simulink model "controllo_test"  (R2020a)
settings: Solver=VariableStepAuto  StartTime=0.0  StopTime=100  RelTol=1e-3
values from neighbouring files (symbols this model uses):
  a = 0.35    [data.m]    (also in geodetic2nedS.m = 6378137)
  a1 = rho * D^4 * alpha1    (= 0.000388302366464)    [data.m]
  a2 = -rho * D^3 * alpha2 * (1 - omega)    (= 0.0037030698432)    [data.m]
  AHRS_bias = [0 0 0]    [data.m]
  AHRS_sample_time = 1/50    (= 0.02)    [data.m]
  AHRS_var = ([1 1 2] * pi/180).^2    [data.m]
  alpha1 = 0.0113    [data.m]
  alpha2 = -0.0091    [data.m]
  c = son2(1)    [Sonar_id.m]    (also in data.m = 0.19)
  current = [seaCurrent; 0; 0; 0]    [data.m]
  D = 0.076    [data.m]
  dead_zone_limit = 31.5    [data.m]
  DVL_sample_t = 1/12    (= 0.0833333333333)    [data.m]
  DVL_var1 = 0.005^2    (= 2.5e-05)    [data.m]
  DVL_var2 = 0.015^2    (= 0.000225)    [data.m]
  DVL_var3 = 0.023^2    (= 0.000529)    [data.m]
  gps_sample_t = 1    [data.m]
  H = eye(3)    [data.m]    (also in navigation_data.m)
  IMU_sample_time = 1/100    (= 0.01)    [data.m]
  initial = []    [data.m]
  INSP = unicode2native(inspectionDirection)    [data.m]
  Ki_bodypos1 = 0    [parametri_PID.m]
  Ki_bodypos2 = 0    [parametri_PID.m]
  Ki_bodypos3 = 0    [parametri_PID.m]
  Ki_bodypos4 = 0    [parametri_PID.m]
  Ki_bodypos5 = 0    [parametri_PID.m]
  Ki_depth1 = 0    [parametri_PID.m]
  Ki_depth2 = 0    [parametri_PID.m]
  Ki_depth3 = 0    [parametri_PID.m]
  Ki_depth4 = 0    [parametri_PID.m]
  Ki_depth5 = 0    [parametri_PID.m]
  Ki_latvel1 = 0    [parametri_PID.m]
  Ki_latvel2 = 0    [parametri_PID.m]
  Ki_latvel3 = 0    [parametri_PID.m]
  Ki_latvel4 = 0    [parametri_PID.m]
  Ki_latvel5 = 0    [parametri_PID.m]
  Ki_P1 = 0    [parametri_PID.m]
  Ki_P2 = 0    [parametri_PID.m]
  Ki_P3 = 0    [parametri_PID.m]
  Ki_P4 = 0    [parametri_PID.m]
  Ki_P5 = 0    [parametri_PID.m]
  Ki_R1 = 0    [parametri_PID.m]
  Ki_R2 = 0    [parametri_PID.m]
  Ki_R3 = 0    [parametri_PID.m]
  Ki_R4 = 0    [parametri_PID.m]
  Ki_R5 = 0    [parametri_PID.m]
  Ki_rel_or1 = 0    [parametri_PID.m]
  Ki_rel_or2 = 0    [parametri_PID.m]
  Ki_rel_or3 = 0    [parametri_PID.m]
  Ki_rel_or4 = 0    [parametri_PID.m]
  Ki_rel_or5 = 0    [parametri_PID.m]
  Ki_reldist1 = 0    [parametri_PID.m]
  Ki_reldist2 = 0    [parametri_PID.m]
  Ki_reldist3 = 0    [parametri_PID.m]
  Ki_reldist4 = 0    [parametri_PID.m]
  Ki_reldist5 = 0    [parametri_PID.m]
  Ki_surge1 = 0    [parametri_PID.m]
  Ki_surge2 = 0    [parametri_PID.m]
  Ki_surge3 = 0    [parametri_PID.m]
  Ki_surge4 = 0    [parametri_PID.m]
  Ki_surge5 = 0    [parametri_PID.m]
  Ki_yaw1 = 0    [parametri_PID.m]
  Ki_yaw2 = 0    [parametri_PID.m]
  Ki_yaw3 = 0    [parametri_PID.m]
  Ki_yaw4 = 0    [parametri_PID.m]
  Ki_yaw5 = 0    [parametri_PID.m]
  Kp_bodypos1 = 0    [parametri_PID.m]
  Kp_bodypos2 = 2    [parametri_PID.m]
  Kp_bodypos3 = 2    [parametri_PID.m]
  Kp_bodypos4 = 2    [parametri_PID.m]
  Kp_bodypos5 = 2    [parametri_PID.m]
  Kp_depth1 = 0    [parametri_PID.m]
  Kp_depth2 = 2    [parametri_PID.m]
  Kp_depth3 = 2    [parametri_PID.m]
  Kp_depth4 = 2    [parametri_PID.m]
  Kp_depth5 = 2    [parametri_PID.m]
  Kp_latvel1 = 0    [parametri_PID.m]
  Kp_latvel2 = 2    [parametri_PID.m]
  Kp_latvel3 = 2    [parametri_PID.m]
  Kp_latvel4 = 2    [parametri_PID.m]
  Kp_latvel5 = 2    [parametri_PID.m]
  Kp_P1 = 0    [parametri_PID.m]
  Kp_P2 = 2    [parametri_PID.m]
  Kp_P3 = 2    [parametri_PID.m]
  Kp_P4 = 2    [parametri_PID.m]
  Kp_P5 = 2    [parametri_PID.m]
  Kp_R1 = 0    [parametri_PID.m]
  Kp_R2 = 2    [parametri_PID.m]
  Kp_R3 = 2    [parametri_PID.m]
  Kp_R4 = 2    [parametri_PID.m]
  Kp_R5 = 2    [parametri_PID.m]
  Kp_rel_or1 = 0    [parametri_PID.m]
  Kp_rel_or2 = 2    [parametri_PID.m]
  Kp_rel_or3 = 2    [parametri_PID.m]
  Kp_rel_or4 = 2    [parametri_PID.m]
  Kp_rel_or5 = 2    [parametri_PID.m]
  Kp_reldist1 = 0    [parametri_PID.m]
  Kp_reldist2 = 2    [parametri_PID.m]
  Kp_reldist3 = 2    [parametri_PID.m]
  Kp_reldist4 = 2    [parametri_PID.m]
  Kp_reldist5 = 2    [parametri_PID.m]
  Kp_surge1 = 0    [parametri_PID.m]
  Kp_surge2 = 2    [parametri_PID.m]
  Kp_surge3 = 2    [parametri_PID.m]
  Kp_surge4 = 2    [parametri_PID.m]
  Kp_surge5 = 2    [parametri_PID.m]
  Kp_yaw1 = 0.6*6    (= 3.6)    [parametri_PID.m]
  Kp_yaw2 = 2    [parametri_PID.m]
  Kp_yaw3 = 2    [parametri_PID.m]
  Kp_yaw4 = 2    [parametri_PID.m]
  Kp_yaw5 = 2    [parametri_PID.m]
  M = M_rb + M_a    [Masse.m]
  M_inv = inv(M)    [Masse.m]
  n_max = 340    [data.m]
  num_cycle = 5    [data.m]    (also in navigation_data.m)
  omega = 0.1    [data.m]
  ps_sample_t = 0.02    [data.m]
  ps_var = (5000/3)^2    (= 2777777.77778)    [data.m]
  pylonCenter = [ 43.723046 ... (first row only)    [missionB.m]
  pylonRadius = 10    [missionB.m]
  ... (+3 more)
undefined symbols (not defined in the file or in its folder): arrival_point, DiscIntNeverNeededParam, Kd_bodypos2, Kd_bodyposy2, Kd_dist_mis2, Kd_surge2, Kd_yaw1, Ki_bodyposy2, Ki_dist_mis2, Kp_dist_mis2, s_data
libraries: simulink x8
(part 4 of 4)

== matlab function controllo_test/Env. & Sensor Model/DVL SENSOR/MATLAB Function ==
  data: ni input; niDVL output; c parameter
function niDVL = traslation(ni, c)
%Calcola la velocità in terna DVL

S = [0,-ni(6),ni(5); 
    ni(6),0,-ni(4); 
    -ni(5),ni(4),0];
p = [0;0;c];
niDVL = ni(1:3,1)+S*p;        %Formula fondamentale della cinematica

== matlab function controllo_test/Vehicle Model/Model Vehicle/D ==
  data: ni_r input; F_d output; rho input
function F_d = D_forces(ni_r, rho)
    ni_lin = ni_r(1:3);
    ni_ang = ni_r(4:6);
    a = 0.35;
    b = a;
    c = 0.19;
    A_ab = pi*a*b;      % moto lin lungo z; rotatorio intorno a x e y
    A_bc = pi*b*c;      % moto lin lungo x; rotatorio intorno a z
    A_ac = pi*a*c;      % moto lin lungo y
%     C_d  =  0.0489;
%     D_coeff = -1/2*rho*C_d*diag([A_bc, A_ac, A_ab, A_bc, A_ac, A_ab]);
%     F_d = D_coeff*(abs(ni_r).*ni_r);
    visc = 0.001;       % Pa*s (per una temperatura di 20° e rho = 1030)
    vmax = 0.3;
    Di = 0.7;
    Re = Di/(visc/rho)*vmax; % Re = 2*1e5
    Cd = 0.49;
    rm_z = 4*c/(3*pi);
    rm_xy = 4*a/(3*pi);
    D_lin = -1/2*rho*Cd*diag([A_bc, A_ac, A_ab])*(abs(ni_lin).*ni_lin);
    D_ang = -1/2*rho*Cd*diag([rm_xy^3*A_ab, rm_xy^3*A_ab, rm_z^3*A_bc])*(abs(ni_ang).*ni_ang);
    F_d = [D_lin; D_ang];
end

== matlab function controllo_test/Env. & Sensor Model/DVL SENSOR/MATLAB Function2 ==
  data: v input; flag output
function flag  = vel_module(v)
%Calcola il modulo della velocità per controllare le condizioni di
%funzionamento del DVL

mod = sqrt((v(1))^2+(v(2))^2+(v(3))^2);

%Da datasheet, se la velocità è superiore ai 9 m/s il sensore non funziona bene
if mod > 9
    flag = 0;
else
    flag = 1;
end
end

== matlab function controllo_test/Controller/AVVICINAMENTO/J2_inv ==
  data: tau_roll input; tau_or_body output; tau_pitch input; tau_yaw input; est_state input
function tau_or_body = fcn(tau_roll,tau_pitch,tau_yaw,est_state)
theta=est_state(1);
phi=est_state(2);
tau_or=[tau_roll;tau_pitch;tau_yaw];
J2_inv = [1       0          -sin(theta); 
         0   cos(phi)  cos(theta)*sin(phi);
         0  -sin(phi)  cos(theta)*cos(phi)];
tau_or_body=J2_inv*tau_or;
end

== matlab function controllo_test/Controller/GEODETIC2NED2/GEODETIC2NED1/MATLAB Function ==
  data: lat input; pos_s_Ned output; lon input
function pos_s_Ned = fcn(lat,lon)
coder.extrinsic('wgs84Ellipsoid','geodetic2ned');
pylonCenter = [43.723046;10.396635];
initPoint = [ 43.722984;10.396204;0];
hOrigin=0;
pos_s_Ned=zeros(3,1);
wgs84=wgs84Ellipsoid('meter');
lat0=pylonCenter(1);
lon0=pylonCenter(2);
h=initPoint(3);
h0=hOrigin;
[xs_N,ys_E,zs_D]=geodetic2ned(lat,lon,h,lat0,lon0,h0,wgs84);
pos_s_Ned=[xs_N,ys_E,zs_D]';
end

== matlab function controllo_test/Env. & Sensor Model/Pressure sensor/MATLAB Function2 ==
  data: h input; p output; rho parameter
function p = pressure(h, rho)
%Calcola la pressione a partire dalla profondità

g = 9.81;                        %accelerazione gravitazionale
p = rho*g*h;
end

== matlab function controllo_test/Env. & Sensor Model/Pressure sensor/MATLAB Function3 ==
  data: orient input; p input; h output; rho parameter; c parameter
function h = depth( orient,  p, rho, c)
%Calcola la profondità misurata dal sensore

phi = orient(1);
theta = orient(2);
psi = orient(3);
Rx_phi = [1 0 0; 0 cos(phi) -sin(phi); 0 sin(phi) cos(phi)];
Ry_theta = [cos(theta) 0 sin(theta); 0 1 0; -sin(theta) 0 cos(theta)];
Rz_psi = [cos(psi) -sin(psi) 0; sin(psi) cos(psi) 0; 0 0 1];

R = Rz_psi*Ry_theta*Rx_phi;
g = 9.81;
cNED = R*[0;0;c];                            %Vettore posizione dell'AUV in terna body riportato in terna NED
h = p/(rho*g)+cNED(3);                       %Il profondimetro è installato sulla pancia dell'AUV, lungo l'asse z
end

== matlab function controllo_test/Controller/GEODETIC2NED3/GEODETIC2NED/MATLAB Function ==
  data: lat input; lon input; pos_Ned output
function pos_Ned = fcn (lat,lon)
coder.extrinsic('wgs84Ellipsoid','geodetic2ned');
pylonCenter = [43.723046;10.396635];
initPoint = [ 43.722984;10.396204;0];
hOrigin=0;
pos_Ned=zeros(3,1)
wgs84=wgs84Ellipsoid('meter')
h=initPoint(3)
lat0=pylonCenter(1)
lon0=pylonCenter(2)
h0=hOrigin
[x_N,y_E,z_D]=geodetic2ned(lat,lon,h,lat,lon,h,wgs84); %TOFIX
pos_Ned=[x_N,y_E,z_D]'
end

== matlab function controllo_test/Controller/IMMERSIONE//RISALITA/J2_inv ==
  data: tau_roll input; tau_or_body output; tau_pitch input; tau_yaw input; est_state input
function tau_or_body = fcn(tau_roll,tau_pitch,tau_yaw,est_state)
theta=est_state(1);
phi=est_state(2);
tau_or=[tau_roll;tau_pitch;tau_yaw];
J2_inv = [1       0          -sin(theta); 
         0   cos(phi)  cos(theta)*sin(phi);
         0  -sin(phi)  cos(theta)*cos(phi)];
tau_or_body=J2_inv*tau_or;
end

== matlab function controllo_test/Env. & Sensor Model/Sonar sensor/MATLAB Function ==
  data: xNorth input; s output; yEast input; zDown input; roll input; pitch input; yaw input; pylonRadius parameter; s_data parameter
function s = Sonar_ideal(xNorth,yEast,zDown,roll,pitch,yaw,pylonRadius, s_data)

coder.extrinsic('Sonar_id');

s_data.num = 5;
s = zeros(s_data.num,1);

s = Sonar_id(xNorth,yEast,zDown,roll,pitch,yaw,pylonRadius,s_data);

== matlab function controllo_test/Vehicle Model/Model Vehicle/C ==
  data: ni_r input; F_c output; M input
function F_c = C(ni_r, M)
    ni = ni_r;
    M11 = M(1:3,1:3);
    M22 = M(4:6,4:6);
    ni1 = ni(1:3);
    ni2 = ni(4:6);
    C11 = zeros(3,3);
    s1 = M11*ni1;
    C12 = - [0 -s1(3) s1(2); s1(3) 0 -s1(1); -s1(2) s1(1) 0];
    C21 = C12;
    s2 = M22*ni2;
    C22 = - [0 -s2(3) s2(2); s2(3) 0 -s2(1); -s2(2) s2(1) 0];
    F_c = [C11 C12; C21 C22]*ni_r;
end

== matlab function controllo_test/Env. & Sensor Model/Sonar sensor/MATLAB Function1 ==
  data: s_in input; s_out output; depth input; error input; flag output; s_data parameter
function [s_out,flag] = Sonar_lim(s_in,depth,error,s_data)
%SONAR_lim
%     [s_out,flag] = Sonar_id[s,error]
%
% Returns the sonar output considering the sensors limitations, but not
% taking into account the bias and error.
%
% flag signals that the corresponding sensor output is affected by
% problems:
% flag += 0     ==>     No errors
% flag += 1     ==>     Under minimum detectable range
% flag += 2     ==>     Over maximum detectable range
% flag += 4     ==>     Over maximum depth
% flag += 8     ==>     Other errors
%
% error is a boolean variable which, when true, sets the flag to += 8

s_data.num = 5;

flag = zeros(s_data.num,1);

s_out = s_in;

for i=1:s_data.num
    if s_in(i) < s_data.minrng
    % Too close
        flag(i) = flag(i)+1;
        s_out(i) = s_data.minrng;
    end
    
    if ( s_in(i) > s_data.maxrng || isnan(s_in(i)) )
    % Too far
        flag(i) = flag(i)+2;
        s_out(i) = NaN;
    end
    
    if depth > s_data.maxdpt
    % Over max depth
        flag(i) = flag(i)+4;
        s_out(i) = NaN;
    end
    
    if error(i) > 0
    % General error flag
        flag(i) = flag(i) + error(i);
        s_out(i) = NaN;
    end
end

end

== matlab function controllo_test/Controller/MATLAB Function1 ==
  data: STATE input; EN output; dist_mis input; yaw_err input; depth_err input; INSP input string
function EN = fcn(STATE,dist_mis,yaw_err,depth_err, INSP)

%EN(1)= bodypos_err
%EN(2)= rel_dist_err
%EN(3)=surge_err
%EN(4)= latvel_err
%EN(5)=depth_err
%EN(6)= RP_err
%EN(7)= rel_or_err
%EN(8)= yaw_err

EN=zeros(1,8)';

if (STATE == 101)
    EN(8)=1;
end
%avvicinamento pilone
if (STATE== 102)
    EN(8)=1;
    EN(3)=1;
    if (STATE==102) && dist_mis<=3.63
        EN(8)=1;
        EN(1)=1;
        EN(3)=0;
    end
end
%rotazione attorno al pilone in superficie
if (STATE == 103)
    EN(2)=1;
    EN(7)=1;
    EN(4)=1;    
    if (yaw_err<=10)
        EN(4)=0;
        EN(8)=1;
        EN(2)=1;
        EN(7)=0;
    end
end
%unicodestr = native2unicode(INSP);
s1=INSP;
s2='vertical';
CMP=strcmp(s1,s2);
if (CMP == 1) %inizio ispezione verticale
    if (STATE==201) 
        EN(2)=1;
        EN(5)=1;
        EN(7)=1;
        EN(6)=1;
        if(depth_err<=3) %stacco i thrusters che controllano la depth
            EN(2)=1;
            EN(7)=1;
            EN(5)=0;
            EN(6)=1;   
        end
    end
    if(STATE==202) && (depth_err<0.2) %controllo di velocità laterale
        EN(2)=1;
        EN(4)=1;
        EN(5)=1;
        EN(6)=1;
        EN(7)=1;
        if(yaw_err<=10) %switch su controllo di posizione
            EN(8)=1;
            EN(2)=1;
            EN(7)=0;
            EN(4)=0; 
            EN(5)=1;
            EN(6)=1;
        end
    end  %fine ispezione verticale
else
    if (STATE==202) && (depth_err<0.2) % inizio ispezione orizzontale
        EN(2)=1;
        EN(5)=1;
        EN(4)=1;  
        EN(7)=1;  
        EN(6)=1;
        if(yaw_err<=10) %switch su controllo di yaw
            EN(8)=1;
            EN(2)=1;
            EN(7)=0; 
            EN(4)=0;
            EN(5)=1;
            EN(6)=1;
        end
    end
    if (STATE==201) %transetto verticale in isp. orizzontale
        EN(2)=1;
        EN(7)=1;
        EN(5)=1;
        EN(6)=1;   
    end 
end     %fine ispezione orizzontale
%fase di immersione   
if(STATE==104)
   EN(2)=1;
   EN(7)=1;
   EN(5)=1;
   EN(6)=1;
   if(depth_err<=3) %stacco i thrusters che controllano la depth
        EN(2)=1;
        EN(7)=1;
        EN(5)=0;
        EN(6)=1;   
   end
end
%fase di risalita
if(STATE==401)
   EN(2)=1;
   EN(7)=1;
   EN(5)=1;
   EN(6)=1;
end   
   
%fase di errore e fine missione
if(STATE == 500) || (STATE == 999)% lascio così poichè in caso di errore
   EN=zeros(1,8)';               % comunque spegnamo tutti i segnali e
                                % lo facciamo risalire attraverso i 4N
end
end

== matlab function controllo_test/Env. & Sensor Model/geodetic2NED1 ==
  data: x output; u input; y output; z output; pylonCenter parameter
function [x, y, z] = fcn(u, pylonCenter)


lat_origin = pylonCenter(1);
lon_origin= pylonCenter(2);
h_origin = pylonCenter(3);

lat=u(1);
lon=u(2);
h=u(3);


[xNorth, yEast, zDown] = geodetic2nedS(lat, lon, h, lat_origin, lon_origin, h_origin);

x = xNorth;
y = yEast;
z = h;

== matlab function controllo_test/Controller/NED2BODY ==
  data: eta1_dot input; mi1 output; phi input; theta input; psi input
function mi1 = fcn(eta1_dot,phi,theta,psi)
Rx_phi=[1 0 0;0 cos(phi) -sin(phi);0 sin(phi) cos(phi)];
Ry_theta=[cos(theta) 0 sin(theta);0 1 0;-sin(theta) 0 cos(theta)];
Rz_psi=[cos(psi) -sin(psi) 0;sin(psi) cos(psi) 0;0 0 1];
J1=Rx_phi*Ry_theta*Rz_psi;
mi1 =J1^-1*eta1_dot;

== matlab function controllo_test/Controller/NED2BODY1 ==
  data: abspos_err input; bodypos_err output; phi input; theta input; psi input
function bodypos_err = fcn(abspos_err,phi,theta,psi)
Rx_phi=   [1      0        0;
           0   cos(phi) -sin(phi);
           0   sin(phi) cos(phi)];
    
Ry_theta=[cos(theta) 0  sin(theta);
              0      1      0;
         -sin(theta) 0  cos(theta)];
     
Rz_psi=  [cos(psi) -sin(psi)  0;
          sin(psi)  cos(psi)  0;
           0           0      1];
       
J1=Rx_phi*Ry_theta*Rz_psi;
bodypos_err=J1^-1*abspos_err

== matlab function controllo_test/Controller/POSIZIONAMENTO/J2_inv ==
  data: tau_roll input; tau_or_body output; tau_pitch input; tau_yaw input; est_state input
function tau_or_body = fcn(tau_roll,tau_pitch,tau_yaw,est_state)
theta=est_state(1);
phi=est_state(2);
tau_or=[tau_roll;tau_pitch;tau_yaw];
J2_inv = [1       0          -sin(theta); 
         0   cos(phi)  cos(theta)*sin(phi);
         0  -sin(phi)  cos(theta)*cos(phi)];
tau_or_body=J2_inv*tau_or;
end

== matlab function controllo_test/Controller/ROTAZIONE IN PROFONDITA'/J2_inv ==
  data: tau_roll input; tau_or_body output; tau_pitch input; tau_yaw input; est_state input
function tau_or_body = fcn(tau_roll,tau_pitch,tau_yaw,est_state)
theta=est_state(1);
phi=est_state(2);
tau_or=[tau_roll;tau_pitch;tau_yaw];
J2_inv = [1       0          -sin(theta); 
         0   cos(phi)  cos(theta)*sin(phi);
         0  -sin(phi)  cos(theta)*cos(phi)];
tau_or_body=J2_inv*tau_or;
end

== matlab function controllo_test/Controller/ROTAZIONE IN SUPERFICIE/J2_inv ==
  data: tau_roll input; tau_or_body output; tau_pitch input; tau_yaw input; est_state input
function tau_or_body = fcn(tau_roll,tau_pitch,tau_yaw,est_state)
theta=est_state(1);
phi=est_state(2);
tau_or=[tau_roll;tau_pitch;tau_yaw];
J2_inv = [1       0          -sin(theta); 
         0   cos(phi)  cos(theta)*sin(phi);
         0  -sin(phi)  cos(theta)*cos(phi)];
tau_or_body=J2_inv*tau_or;
end

== matlab function controllo_test/Vehicle Model/Model Vehicle/grav ==
  data: rho input; eta input; F_g output
function F_g = grav(rho, eta)
    eta2 = eta(4:6);
    g = 9.81;   
    a = 0.35;
    b = a;
    c = 0.19;
    massa = 100;
    if eta(3) >= c
       V = 4/3*pi*a*b*c;
    else
       V = 4/3*pi*a*b*c - (pi*a*b/(3*c^2))*((eta(3)-c)^2)*(3*c - abs(eta(3) - c)); 
    end
    W = massa*g;
    B = rho*V*g;
    J = Jac(eta2);
    J1 = J(1:3,1:3);
    J2 = J(4:6,4:6);
    f_g = inv(J1)*[0; 0; W];
    f_b = inv(J1)*[0; 0; -B];
    r_g = [0; 0; 0];
    r_b = [0; 0; -c/2];
    %TODO: inserire un contributo nullo di forza quando siamo a galla (?)
%     if eta(3) < 0
%        F_g = [0; 0; 0; 0; 0; 0];
%     else
    F_g = -[f_g + f_b; cross(r_g,f_g) + cross(r_b,f_b)];
%     end
end

== matlab function controllo_test/Controller/T2n/MATLAB Function ==
  data: Tdes input; n output
function n  = fcn(Tdes)
n=zeros(1,7)';
a1=0.000388302366464000;
%assunzione modello a bassa velocità
for i=1:1:7
       n(i)=sign(Tdes(i))*sqrt((abs(Tdes(i))/a1));  
end
end

== matlab function controllo_test/Controller/Tau2T/Tau2T ==
  data: tau_des input; T output
function T= fcn(tau_des)
p1 = [0 -0.25 0]';
p2 = [0 0.25 0]';
p3 = [-0.25 0 0]';
p4 = [0.25 0 0]';
p5 = [-0.15 -0.15 0]';
p6 = [-0.15 0.15 0]';
p7 = [0.15 0 0]';

t1 = [1 0 0]';
t2 = t1;
t3 = [0 1 0]';
t4 = -t3;
t5 = [0 0 1]';
t6 = t5;
t7 = t5;

B1 = [t1; cross(p1,t1)];
B2 = [t2; cross(p2,t2)];
B3 = [t3; cross(p3,t3)];
B4 = [t4; cross(p4,t4)];
B5 = [t5; cross(p5,t5)];
B6 = [t6; cross(p6,t6)];
B7 = [t7; cross(p7,t7)];
B = [B1 B2 B3 B4 B5 B6 B7];

Bpinv=pinv(B);
T = Bpinv*tau_des;

end

== matlab function controllo_test/Controller/Tau2T/Tau_des ENABLE ==
  data: STATE input; tau_des output; tau1 input; tau2 input; tau3 input; tau4 input; tau5 input
function tau_des= fcn(STATE,tau1,tau2,tau3,tau4,tau5)
tau_des= zeros(1,6)';
if (STATE==101)
    tau_des=tau1;
end
if (STATE==102)
    tau_des=tau2;
end
if (STATE==103)
    tau_des= tau3;
end
if (STATE== 201|| STATE==104||STATE==401)
    tau_des=tau4;
end
if (STATE== 202)
    tau_des=tau5;
end
if (STATE==500 || STATE== 999)
    tau_des=zeros(1,6)';
end
end

== matlab function controllo_test/Controller/wrapTopi ==
  data: u input; y output
function y = fcn(u)
coder.extrinsic('wrapToPi');
y=0;
y = wrapToPi(u);
end

== matlab function controllo_test/Controller/wrapTopi1 ==
  data: u input; y output
function y = fcn(u)
coder.extrinsic('wrapToPi');
y=0;
y = wrapToPi(u);
end

== matlab function controllo_test/Navigation1/Relative estimation/flag_sonar_func ==
  data: flag_sonar input; flag output; s_data parameter
function flag = fcn(flag_sonar, s_data)

flag = 1;

if sum(flag_sonar) >= (s_data.num-1)*8
    flag = 0;
else 
    flag = 1;
end

== matlab function controllo_test/Controller/MATLAB Function ==
  data: u input; dist_mis output; arrival_point input
function dist_mis = fcn(u,arrival_point)
dist_mis=sqrt((arrival_point(1)-u(1))^2+(arrival_point(2)-u(2))^2);

== matlab function controllo_test/Vehicle Model/Model Vehicle/Kinematic/Jac ==
  data: eta input; J output
function J = Jac(eta)
    eta2 = eta(4:6);
    phi = eta2(1);
    theta = eta2(2);
    psi = eta2(3);
    Rx = [1 0 0; 0 cos(phi) sin(phi); 0 -sin(phi) cos(phi)];
    Ry = [cos(theta) 0 -sin(theta); 0 1 0; sin(theta) 0 cos(theta)];
    Rz = [cos(psi) sin(psi) 0; -sin(psi) cos(psi) 0; 0 0 1];
    J1 = Rz'*Ry'*Rx';
    J2 = [1 sin(phi)*tan(theta) cos(phi)*tan(theta); ...
        0 cos(phi) -sin(phi); ...
        0 sin(phi)/cos(theta) cos(phi)/cos(theta)];
    J = blkdiag(J1, J2);
end

== matlab function controllo_test/Vehicle Model/Thrusters/T/Thruster 1/MATLAB Function ==
  data: n input; T output; V input; D parameter; omega parameter; a1 parameter; a2 parameter; alpha1 parameter; alpha2 parameter
function T = thrusterModel(n, V, D, omega, a1, a2, alpha1, alpha2)

Va = (1-omega) * V;     % Advancement velocity at the propeller
J0 = Va/(n*D);          % Advancement Coefficient

if J0 > -alpha1/alpha2  % Out of linearity domain (right side)
    T = 0;              % A null generated thrust is assumed
    
elseif J0 < 0           % Out of linearity domain (left side)
    T = a1*abs(n)*n;    % Bollard thrust is assumed

else                    % Within the linearity domain
    T = a1*abs(n)*n - a2*abs(n)*V;
end

== matlab function controllo_test/Vehicle Model/Thrusters/T/Thruster 2/MATLAB Function ==
  data: n input; T output; V input; D parameter; omega parameter; a1 parameter; a2 parameter; alpha1 parameter; alpha2 parameter
function T = thrusterModel(n, V, D, omega, a1, a2, alpha1, alpha2)

Va = (1-omega) * V;     % Advancement velocity at the propeller
J0 = Va/(n*D);          % Advancement Coefficient

if J0 > -alpha1/alpha2  % Out of linearity domain (right side)
    T = 0;              % A null generated thrust is assumed
    
elseif J0 < 0           % Out of linearity domain (left side)
    T = a1*abs(n)*n;    % Bollard thrust is assumed

else                    % Within the linearity domain
    T = a1*abs(n)*n - a2*abs(n)*V;
end
